simulink model "digital"  (R2025a)
settings: Solver=VariableStepAuto  StartTime=0.0  StopTime=10.0  RelTol=1e-3
settings Model: Creator=joasb  LastModifiedBy=joasb

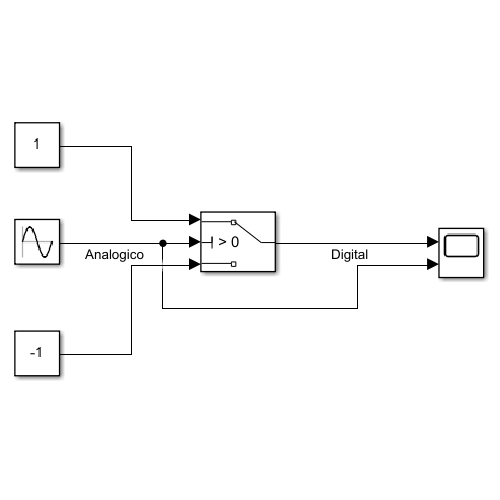
[thumbnail: Simulink's stored preview of the top-level diagram]
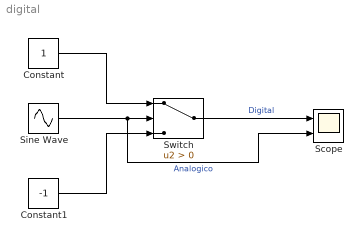
== system digital ==
  Constant : Constant
  Constant1 : Constant  Value=-1
  Scope : Scope  NumInputPorts=2
      settings: ActiveDisplayYMinimum=-1.2494670038018805  ActiveDisplayYMaximum=1.2494670038018814
  Sine Wave : Sin  SampleTime=0
  Switch : Switch  Criteria=u2 > Threshold  SaturateOnIntegerOverflow=off  InputSameDT=off
  wires:
  Sine Wave/1 -> Scope/2, Switch/2  "Analogico"
  Constant/1 -> Switch/1
  Constant1/1 -> Switch/3
  Switch/1 -> Scope/1  "Digital"
